simulink library "bpm_blower_propulsion_module_lib"  (R2015b)
settings: Solver=ode45  StartTime=0.0  StopTime=10.0  RelTol=1e-3
values from neighbouring files (symbols this model uses):
  bpm_imp_cmd_filt_den = single(1.0)    [bpm_blower_propulsion_module_init.m]
  bpm_imp_cmd_filt_num = single(1.0)    [bpm_blower_propulsion_module_init.m]
  bpm_imp_ctl_filt_n = single(1.0)    [bpm_blower_propulsion_module_init.m]
  bpm_imp_ctl_kd = single(0.001)    [bpm_blower_propulsion_module_init.m]
  bpm_imp_ctl_ki = single(0.40)    [bpm_blower_propulsion_module_init.m]
  bpm_imp_ctl_kp = single(0.015)    [bpm_blower_propulsion_module_init.m]
  bpm_imp_ctl_ts = 0.016    [bpm_blower_propulsion_module_init.m]
  bpm_imp_max_voltage = single(16.6)    [bpm_blower_propulsion_module_init.m]
  bpm_imp_motor_friction_coeff = bpm_imp_noload_curr*bpm_imp_motor_torque_k/bpm_imp_noload_speed    [bpm_blower_propulsion_module_prep.m]
  bpm_imp_motor_r = single(1.2)    [bpm_blower_propulsion_module_init.m]
  bpm_imp_motor_speed_k = single(374*2*pi/60)    [bpm_blower_propulsion_module_init.m]
  bpm_imp_motor_torque_k = single(0.0255)    [bpm_blower_propulsion_module_init.m]
  bpm_imp_speed_filt_den = single(1.0)    [bpm_blower_propulsion_module_init.m]
  bpm_imp_speed_filt_num = single(1.0)    [bpm_blower_propulsion_module_init.m]
  bpm_sensor_delay = 1    [bpm_blower_propulsion_module_init.m]
  bpm_sensor_rand_seed = 1337    [bpm_blower_propulsion_module_init.m]
  bpm_sensor_sf = single(1)    [bpm_blower_propulsion_module_init.m]
  bpm_sensor_sigma_u = .00001    (= 1e-05)    [bpm_blower_propulsion_module_init.m]
  bpm_sensor_sigma_v = .00001    (= 1e-05)    [bpm_blower_propulsion_module_init.m]
  bpm_servo_ctl_filt_n = single(1.0)    [bpm_blower_propulsion_module_init.m]
  bpm_servo_ctl_kd = single(0.8)    [bpm_blower_propulsion_module_init.m]
  bpm_servo_ctl_ki = single(1.5)    [bpm_blower_propulsion_module_init.m]
  bpm_servo_ctl_kp = single(5.0)    [bpm_blower_propulsion_module_init.m]
  bpm_servo_ctl_ts = 0.016    [bpm_blower_propulsion_module_init.m]
  bpm_servo_max_theta = abp_nozzle_gear_ratio*(abp_nozzle_max_open_angle - abp_nozzle_min_open_angle)    [bpm_blower_propulsion_module_prep.m]
  bpm_servo_max_voltage = single(6)    [bpm_blower_propulsion_module_init.m]
  bpm_servo_min_theta = 0    [bpm_blower_propulsion_module_prep.m]
  bpm_servo_motor_friction_coeff = single(0.0000003)    [bpm_blower_propulsion_module_init.m]
  bpm_servo_motor_gear_box_inertia = single(.000000025)    [bpm_blower_propulsion_module_init.m]
  bpm_servo_motor_gear_ratio = single(1/100)    [bpm_blower_propulsion_module_init.m]
  bpm_servo_motor_k = bpm_servo_peak_torque*bpm_servo_motor_gear_ratio/(bpm_servo_peak_curr)    [bpm_blower_propulsion_module_prep.m]
  bpm_servo_motor_r = bpm_servo_max_voltage/bpm_servo_peak_curr    [bpm_blower_propulsion_module_prep.m]
  bpm_servo_pwm2angle = (bpm_servo_max_theta-bpm_servo_min_theta)/(abp_servo_max_PWM-abp_servo_min_PWM)    [bpm_blower_propulsion_module_prep.m]
  bpm_servo_pwm2angle_bias = bpm_servo_min_theta/bpm_servo_pwm2angle - abp_servo_min_PWM    [bpm_blower_propulsion_module_prep.m]
undefined symbols (not defined in the file or in its folder): astrobee_time_step_size, bpm_blower_speed2pwm, bpm_nozzle_gear_ratio, DiscIntNeverNeededParam
libraries: bpm_common_lib x4, simulink x3, util_common_lib x1
settings Model: Creator=rhnakamu  LastModifiedBy=jfusco1
settings DataIOCC: SaveFormat=Array
settings HardwareCC: ProdBitPerPointer=32  ProdLargestAtomicFloat=None  ProdIntDivRoundTo=Undefined  ProdEndianess=Unspecified  ProdWordSize=32  ProdHWDeviceType=32-bit Generic
settings GRTTargetCC: GeneratePreprocessorConditionals=Disable all
settings ConfigComp: CovModelRefEnable=Off

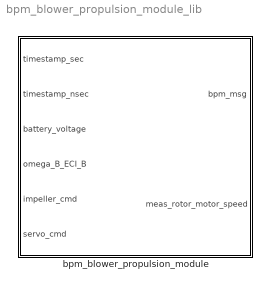
== system bpm_blower_propulsion_module_lib ==
  bpm_blower_propulsion_module : Subsystem

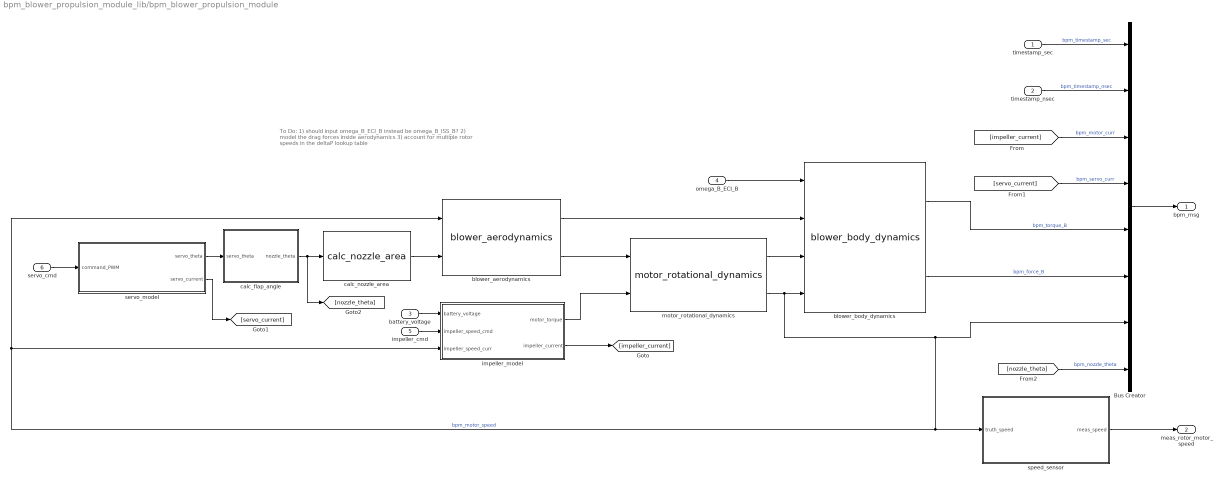
== system bpm_blower_propulsion_module_lib/bpm_blower_propulsion_module ==
  note: To Do:
      | 	1) should input omega_B_ECI_B instead be omega_B_ISS_B?
      | 	2) model the drag forces inside aerodynamics
      | 	3) account for multiple rotor speeds in the deltaP lookup table
  timestamp_sec : Inport
  timestamp_nsec : Inport  Port=2
  battery_voltage : Inport  Port=3
  omega_B_ECI_B : Inport  Port=4
  impeller_cmd : Inport  Port=5
  servo_cmd : Inport  Port=6
  Bus Creator : BusCreator  Inputs=8  OutDataTypeStr=Bus: bpm_msg  NonVirtualBus=on
      settings: InheritFromInputs=off
  blower_aerodynamics : bpm_common_lib/blower_aerodynamics  VariantControl=blw_blower_algebraic == true
  blower_body_dynamics : bpm_common_lib/blower_body_dynamics
  calc_flap_angle : Subsystem
  calc_nozzle_area : bpm_common_lib/calc_nozzle_area
  impeller_model : Subsystem
  motor_rotational_dynamics : bpm_common_lib/motor_rotational_dynamics
  servo_model : Subsystem  TreatAsAtomicUnit=on
  speed_sensor : Subsystem
  bpm_msg : Outport
  meas_rotor_motor_speed : Outport  Port=2
  wires:
  timestamp_sec/1 -> Bus Creator/1  "bpm_timestamp_sec"
  timestamp_nsec/1 -> Bus Creator/2  "bpm_timestamp_nsec"
  [nozzle_theta] -> Bus Creator/8  "bpm_nozzle_theta"
  blower_aerodynamics/1 -> blower_body_dynamics/2
  battery_voltage/1 -> impeller_model/1(battery_voltage)
  servo_model/1(servo_theta) -> calc_flap_angle/1(servo_theta)
  calc_nozzle_area/1 -> blower_aerodynamics/2
  motor_rotational_dynamics/2 -> blower_body_dynamics/4, blower_aerodynamics/1, impeller_model/3(impeller_speed_curr), speed_sensor/1(truth_speed), Bus Creator/7  "bpm_motor_speed"
  servo_model/2(servo_current) -> [servo_current]
  blower_body_dynamics/1 -> Bus Creator/5  "bpm_torque_B"
  blower_body_dynamics/2 -> Bus Creator/6  "bpm_force_B"
  speed_sensor/1(meas_speed) -> meas_rotor_motor_speed/1
  omega_B_ECI_B/1 -> blower_body_dynamics/1
  servo_cmd/1 -> servo_model/1(command_PWM)
  impeller_cmd/1 -> impeller_model/2(impeller_speed_cmd)
  impeller_model/1(motor_torque) -> motor_rotational_dynamics/2
  impeller_model/2(impeller_current) -> [impeller_current]
  [servo_current] -> Bus Creator/4  "bpm_servo_curr"
  [impeller_current] -> Bus Creator/3  "bpm_motor_curr"
  Bus Creator/1 -> bpm_msg/1
  calc_flap_angle/1(nozzle_theta) -> [nozzle_theta], calc_nozzle_area/1
  blower_aerodynamics/2 -> motor_rotational_dynamics/1
  motor_rotational_dynamics/1 -> blower_body_dynamics/3

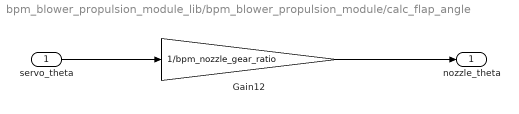
== system bpm_blower_propulsion_module_lib/bpm_blower_propulsion_module/calc_flap_angle ==
  servo_theta : Inport
  Gain12 : Gain  Gain=1/bpm_nozzle_gear_ratio
  nozzle_theta : Outport
  wires:
  servo_theta/1 -> Gain12/1
  Gain12/1 -> nozzle_theta/1

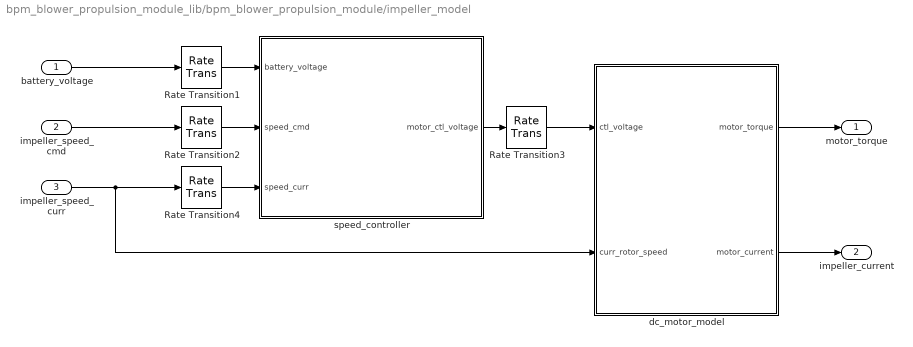
== system bpm_blower_propulsion_module_lib/bpm_blower_propulsion_module/impeller_model ==
  battery_voltage : Inport
  impeller_speed_cmd : Inport  Port=2
  impeller_speed_curr : Inport  Port=3
  Rate Transition{1..4} (4 alike) : RateTransition
      settings: AttributesFormatString=sampleTime: %<OutPortSampleTime>
  dc_motor_model : Subsystem  TreatAsAtomicUnit=on
  speed_controller : Subsystem  TreatAsAtomicUnit=on
  motor_torque : Outport
  impeller_current : Outport  Port=2
  wires:
  impeller_speed_cmd/1 -> Rate Transition2/1
  Rate Transition4/1 -> speed_controller/3(speed_curr)
  Rate Transition2/1 -> speed_controller/2(speed_cmd)
  Rate Transition1/1 -> speed_controller/1(battery_voltage)
  Rate Transition3/1 -> dc_motor_model/1(ctl_voltage)
  battery_voltage/1 -> Rate Transition1/1
  dc_motor_model/2(motor_current) -> impeller_current/1
  speed_controller/1(motor_ctl_voltage) -> Rate Transition3/1
  dc_motor_model/1(motor_torque) -> motor_torque/1
  impeller_speed_curr/1 -> dc_motor_model/2(curr_rotor_speed), Rate Transition4/1

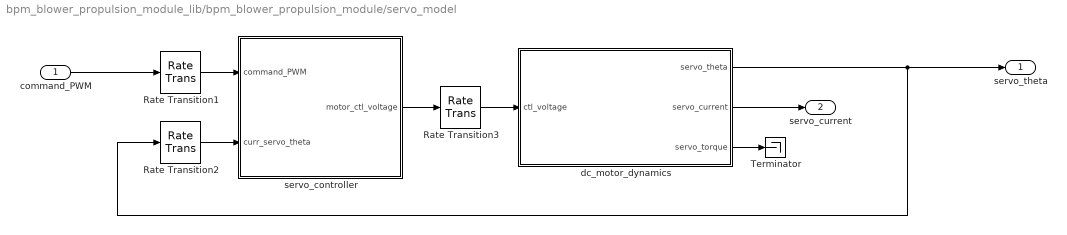
== system bpm_blower_propulsion_module_lib/bpm_blower_propulsion_module/servo_model ==
  command_PWM : Inport
  Rate Transition1 : RateTransition
      settings: AttributesFormatString=sampleTime: %<OutPortSampleTime>
  Rate Transition2 : RateTransition
      settings: AttributesFormatString=sampleTime: %<OutPortSampleTime>
  Rate Transition3 : RateTransition
      settings: AttributesFormatString=sampleTime: %<OutPortSampleTime>
  Terminator : Terminator
  dc_motor_dynamics : Subsystem
  servo_controller : Subsystem
  servo_theta : Outport
  servo_current : Outport  Port=2
  wires:
  dc_motor_dynamics/3(servo_torque) -> Terminator/1
  command_PWM/1 -> Rate Transition1/1
  servo_controller/1(motor_ctl_voltage) -> Rate Transition3/1
  Rate Transition3/1 -> dc_motor_dynamics/1(ctl_voltage)
  Rate Transition1/1 -> servo_controller/1(command_PWM)
  Rate Transition2/1 -> servo_controller/2(curr_servo_theta)
  dc_motor_dynamics/2(servo_current) -> servo_current/1
  dc_motor_dynamics/1(servo_theta) -> servo_theta/1, Rate Transition2/1

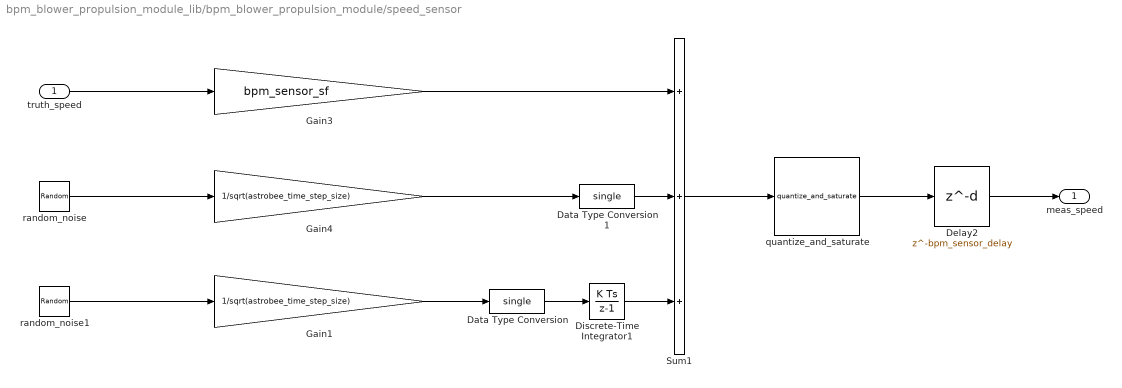
== system bpm_blower_propulsion_module_lib/bpm_blower_propulsion_module/speed_sensor ==
  truth_speed : Inport
  Data Type Conversion : DataTypeConversion  OutDataTypeStr=single
  Data Type Conversion1 : DataTypeConversion  OutDataTypeStr=single
  Delay2 : Delay  DelayLength=bpm_sensor_delay
      settings: AttributesFormatString=|
      | IC: %<InitialCondition>
      | Delay: %<DelayLength>
  Discrete-Time Integrator1 : DiscreteIntegrator  InitialCondition=single(0)  InitialConditionSetting=State (most efficient)  SampleTime=-1  ICPrevOutput=DiscIntNeverNeededParam  ICPrevScaledInput=DiscIntNeverNeededParam
      settings: AttributesFormatString=IC:%<InitialCondition>
  Gain1 : Gain  Gain=1/sqrt(astrobee_time_step_size)
  Gain3 : Gain  Gain=bpm_sensor_sf
  Gain4 : Gain  Gain=1/sqrt(astrobee_time_step_size)
  Sum1 : Sum  Inputs=+++
  quantize_and_saturate : util_common_lib/quantize_and_saturate  RES=bpm_sensor_resolution  OPER=truncate  out_min=bpm_sensor_min  out_max=bpm_sensor_max
      settings: AttributesFormatString=|
      | Resolution: %<RES>
      | Max: %<out_max>
      | Min: %<out_min>
  random_noise : RandomNumber  Variance=bpm_sensor_sigma_u.^2  Seed=bpm_sensor_rand_seed  SampleTime=astrobee_time_step_size
      settings: AttributesFormatString=|
      | Variance:%<Variance>
      | Mean:%<Mean>
      | Seed:%<Seed>
      | Sample Time:%<SampleTime>
  random_noise1 : RandomNumber  Variance=bpm_sensor_sigma_v.^2  Seed=bpm_sensor_rand_seed+1  SampleTime=astrobee_time_step_size
      settings: AttributesFormatString=|
      | Variance:%<Variance>
      | Mean:%<Mean>
      | Seed:%<Seed>
      | Sample Time:%<SampleTime>
  meas_speed : Outport
  wires:
  Data Type Conversion/1 -> Discrete-Time Integrator1/1
  Gain3/1 -> Sum1/1
  Data Type Conversion1/1 -> Sum1/2
  Discrete-Time Integrator1/1 -> Sum1/3
  Sum1/1 -> quantize_and_saturate/1
  Gain4/1 -> Data Type Conversion1/1
  Gain1/1 -> Data Type Conversion/1
  random_noise1/1 -> Gain1/1
  random_noise/1 -> Gain4/1
  truth_speed/1 -> Gain3/1
  quantize_and_saturate/1 -> Delay2/1
  Delay2/1 -> meas_speed/1

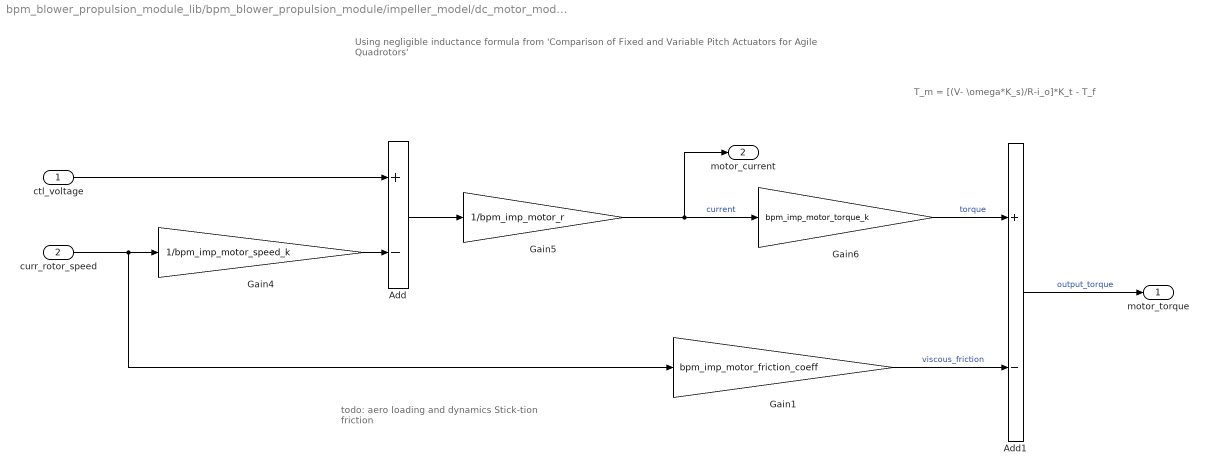
== system bpm_blower_propulsion_module_lib/bpm_blower_propulsion_module/impeller_model/dc_motor_model ==
  note: todo:
      | aero loading and dynamics
      | Stick-tion friction
  note: Using negligible inductance formula from 'Comparison of Fixed and Variable Pitch Actuators for Agile Quadrotors'
  note: T_m = [(V- \omega*K_s)/R-i_o]*K_t - T_f
  ctl_voltage : Inport
  curr_rotor_speed : Inport  Port=2
  Add : Sum  Inputs=+-
  Add1 : Sum  Inputs=+-
  Gain1 : Gain  Gain=bpm_imp_motor_friction_coeff
  Gain4 : Gain  Gain=1/bpm_imp_motor_speed_k
  Gain5 : Gain  Gain=1/bpm_imp_motor_r
  Gain6 : Gain  Gain=bpm_imp_motor_torque_k
  motor_torque : Outport
  motor_current : Outport  Port=2
  wires:
  Gain5/1 -> Gain6/1, motor_current/1  "current"
  ctl_voltage/1 -> Add/1
  Gain4/1 -> Add/2
  curr_rotor_speed/1 -> Gain1/1, Gain4/1
  Add/1 -> Gain5/1
  Gain6/1 -> Add1/1  "torque"
  Add1/1 -> motor_torque/1  "output_torque"
  Gain1/1 -> Add1/2  "viscous_friction"

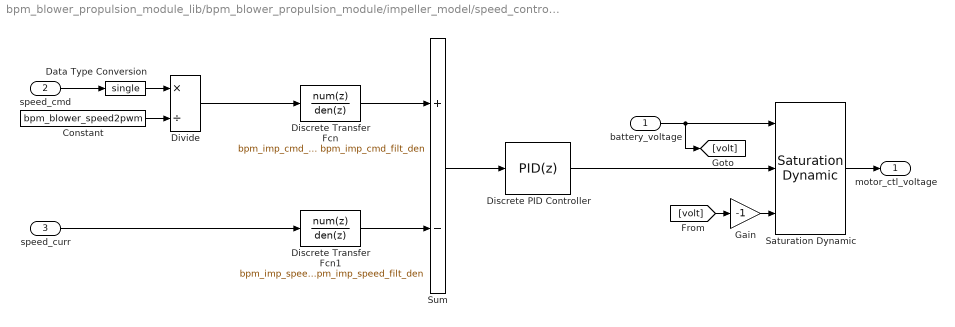
== system bpm_blower_propulsion_module_lib/bpm_blower_propulsion_module/impeller_model/speed_controller ==
  battery_voltage : Inport
  speed_cmd : Inport  Port=2
  speed_curr : Inport  Port=3
  Constant : Constant  Value=bpm_blower_speed2pwm
  Data Type Conversion : DataTypeConversion  OutDataTypeStr=single
  Discrete Transfer Fcn : DiscreteTransferFcn  Numerator=bpm_imp_cmd_filt_num  Denominator=bpm_imp_cmd_filt_den  SampleTime=bpm_imp_ctl_ts
      settings: AttributesFormatString=|
      | Num: %<Numerator>
      | Den: %<Denominator>
      | TS: %<SampleTime>
  Discrete Transfer Fcn1 : DiscreteTransferFcn  Numerator=bpm_imp_speed_filt_num  Denominator=bpm_imp_speed_filt_den  SampleTime=bpm_imp_ctl_ts
      settings: AttributesFormatString=|
      | Num: %<Numerator>
      | Den: %<Denominator>
      | TS: %<SampleTime>
  Discrete PID Controller : simulink/Continuous/PID Controller  Controller=PID  TimeDomain=Discrete-time  SampleTime=bpm_imp_ctl_ts  IntegratorMethod=Forward Euler  FilterMethod=Forward Euler  Form=Parallel  UseFilter=on  ControllerParametersSource=internal  P=bpm_imp_ctl_kp  I=bpm_imp_ctl_ki  D=bpm_imp_ctl_kd  N=bpm_imp_ctl_filt_n  InitialConditionSource=internal  InitialConditionForIntegrator=0  InitialConditionForFilter=0  ExternalReset=none  LimitOutput=on  UpperSaturationLimit=bpm_imp_max_voltage  LowerSaturationLimit=-bpm_imp_max_voltage  LinearizeAsGain=off  AntiWindupMode=clamping  Kb=1  TrackingMode=off  Kt=1  PParamMin=[]  PParamMax=[]  IParamMin=[]  IParamMax=[]  DParamMin=[]  DParamMax=[]  NParamMin=[]  NParamMax=[]  KbParamMin=[]  KbParamMax=[]  KtParamMin=[]  KtParamMax=[]  POutMin=[]  POutMax=[]  IOutMin=[]  IOutMax=[]  DOutMin=[]  DOutMax=[]  NOutMin=[]  NOutMax=[]  KbOutMin=[]  KbOutMax=[]  KtOutMin=[]  KtOutMax=[]  IntegratorOutMin=[]  IntegratorOutMax=[]  FilterOutMin=[]  FilterOutMax=[]  SumOutMin=[]  SumOutMax=[]  SumI1OutMin=[]  SumI1OutMax=[]  SumI2OutMin=[]  SumI2OutMax=[]  SumI3OutMin=[]  SumI3OutMax=[]  SumDOutMin=[]  SumDOutMax=[]  SaturationOutMin=[]  SaturationOutMax=[]  IntegratorContinuousStateAttributes=''  IntegratorStateMustResolveToSignalObject=off  IntegratorRTWStateStorageClass=Auto  FilterContinuousStateAttributes=''  FilterStateMustResolveToSignalObject=off  FilterRTWStateStorageClass=Auto  DifferentiatorICPrevScaledInput=0  DifferentiatorOutMin=[]  DifferentiatorOutMax=[]
      settings: AttributesFormatString=|
      | Kp: %<P>
      | Ki: %<I>
      | Kd: %<D>
      | NFilt: %<N>
      | Ts: %<SampleTime>
      | 
      | min: %<LowerSaturationLimit>
      | max: %<UpperSaturationLimit>
  Divide : Product  Inputs=*/
  Gain : Gain  Gain=-1
  Saturation Dynamic : simulink/Discontinuities/Saturation Dynamic  OutMin=[]  OutMax=[]  OutDataTypeStr=Inherit: Same as second input  OutDataType=fixdt(1, 16)  OutScaling=2^-10  DoSatur=off
  Sum : Sum  Inputs=+-
  motor_ctl_voltage : Outport
  wires:
  Gain/1 -> Saturation Dynamic/3
  [volt] -> Gain/1
  Discrete PID Controller/1 -> Saturation Dynamic/2
  battery_voltage/1 -> [volt], Saturation Dynamic/1
  speed_curr/1 -> Discrete Transfer Fcn1/1
  Sum/1 -> Discrete PID Controller/1
  Saturation Dynamic/1 -> motor_ctl_voltage/1
  Discrete Transfer Fcn1/1 -> Sum/2
  Discrete Transfer Fcn/1 -> Sum/1
  speed_cmd/1 -> Data Type Conversion/1
  Divide/1 -> Discrete Transfer Fcn/1
  Constant/1 -> Divide/2
  Data Type Conversion/1 -> Divide/1

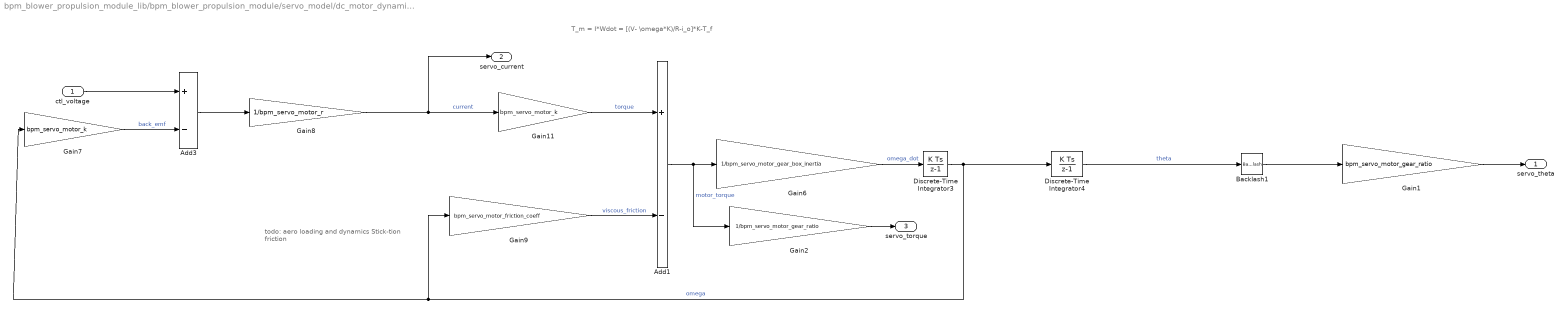
== system bpm_blower_propulsion_module_lib/bpm_blower_propulsion_module/servo_model/dc_motor_dynamics ==
  note: T_m = I*Wdot = [(V- \omega*K)/R-i_o]*K-T_f
  note: todo:
      | aero loading and dynamics
      | Stick-tion friction
  ctl_voltage : Inport
  Add1 : Sum  Inputs=+-
  Add3 : Sum  Inputs=+-
  Backlash1 : Backlash  BacklashWidth=bpm_servo_motor_backlash_deadband
      settings: AttributesFormatString=width: %<BacklashWidth>
  Discrete-Time Integrator3 : DiscreteIntegrator  InitialCondition=single(0)  SampleTime=-1  ICPrevOutput=DiscIntNeverNeededParam  ICPrevScaledInput=DiscIntNeverNeededParam
      settings: AttributesFormatString=IC: %<InitialCondition>
  Discrete-Time Integrator4 : DiscreteIntegrator  InitialCondition=bpm_servo_min_theta/bpm_servo_motor_gear_ratio  SampleTime=-1  LimitOutput=on  UpperSaturationLimit=bpm_servo_max_theta/bpm_servo_motor_gear_ratio  LowerSaturationLimit=bpm_servo_min_theta/bpm_servo_motor_gear_ratio  ICPrevOutput=DiscIntNeverNeededParam  ICPrevScaledInput=DiscIntNeverNeededParam
      settings: AttributesFormatString=|
      | IC: %<InitialCondition>
      | max: %<UpperSaturationLimit>
      | min: %<LowerSaturationLimit>
  Gain1 : Gain  Gain=bpm_servo_motor_gear_ratio
  Gain11 : Gain  Gain=bpm_servo_motor_k
  Gain2 : Gain  Gain=1/bpm_servo_motor_gear_ratio
  Gain6 : Gain  Gain=1/bpm_servo_motor_gear_box_inertia
  Gain7 : Gain  Gain=bpm_servo_motor_k
  Gain8 : Gain  Gain=1/bpm_servo_motor_r
  Gain9 : Gain  Gain=bpm_servo_motor_friction_coeff
  servo_theta : Outport
  servo_current : Outport  Port=2
  servo_torque : Outport  Port=3
  wires:
  ctl_voltage/1 -> Add3/1
  Gain2/1 -> servo_torque/1
  Gain9/1 -> Add1/2  "viscous_friction"
  Gain11/1 -> Add1/1  "torque"
  Add1/1 -> Gain2/1, Gain6/1  "motor_torque"
  Gain1/1 -> servo_theta/1
  Backlash1/1 -> Gain1/1
  Discrete-Time Integrator3/1 -> Gain9/1, Gain7/1, Discrete-Time Integrator4/1  "omega"
  Discrete-Time Integrator4/1 -> Backlash1/1  "theta"
  Gain8/1 -> servo_current/1, Gain11/1  "current"
  Add3/1 -> Gain8/1
  Gain7/1 -> Add3/2  "back_emf"
  Gain6/1 -> Discrete-Time Integrator3/1  "omega_dot"

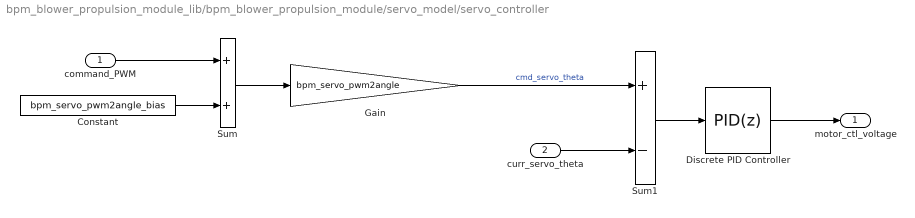
== system bpm_blower_propulsion_module_lib/bpm_blower_propulsion_module/servo_model/servo_controller ==
  command_PWM : Inport
  curr_servo_theta : Inport  Port=2
  Constant : Constant  Value=bpm_servo_pwm2angle_bias
  Discrete PID Controller : simulink/Continuous/PID Controller  Controller=PID  TimeDomain=Discrete-time  SampleTime=bpm_servo_ctl_ts  IntegratorMethod=Forward Euler  FilterMethod=Forward Euler  Form=Parallel  UseFilter=on  ControllerParametersSource=internal  P=bpm_servo_ctl_kp  I=bpm_servo_ctl_ki  D=bpm_servo_ctl_kd  N=bpm_servo_ctl_filt_n  InitialConditionSource=internal  InitialConditionForIntegrator=0  InitialConditionForFilter=0  ExternalReset=none  LimitOutput=on  UpperSaturationLimit=bpm_servo_max_voltage  LowerSaturationLimit=-bpm_servo_max_voltage  LinearizeAsGain=off  AntiWindupMode=clamping  Kb=1  TrackingMode=off  Kt=1  PParamMin=[]  PParamMax=[]  IParamMin=[]  IParamMax=[]  DParamMin=[]  DParamMax=[]  NParamMin=[]  NParamMax=[]  KbParamMin=[]  KbParamMax=[]  KtParamMin=[]  KtParamMax=[]  POutMin=[]  POutMax=[]  IOutMin=[]  IOutMax=[]  DOutMin=[]  DOutMax=[]  NOutMin=[]  NOutMax=[]  KbOutMin=[]  KbOutMax=[]  KtOutMin=[]  KtOutMax=[]  IntegratorOutMin=[]  IntegratorOutMax=[]  FilterOutMin=[]  FilterOutMax=[]  SumOutMin=[]  SumOutMax=[]  SumI1OutMin=[]  SumI1OutMax=[]  SumI2OutMin=[]  SumI2OutMax=[]  SumI3OutMin=[]  SumI3OutMax=[]  SumDOutMin=[]  SumDOutMax=[]  SaturationOutMin=[]  SaturationOutMax=[]  IntegratorContinuousStateAttributes=''  IntegratorStateMustResolveToSignalObject=off  IntegratorRTWStateStorageClass=Auto  FilterContinuousStateAttributes=''  FilterStateMustResolveToSignalObject=off  FilterRTWStateStorageClass=Auto  DifferentiatorICPrevScaledInput=0  DifferentiatorOutMin=[]  DifferentiatorOutMax=[]
      settings: AttributesFormatString=|
      | Kp: %<P>
      | Ki: %<I>
      | Kd: %<D>
      | NFilt: %<N>
      | Ts: %<SampleTime>
      | 
      | Min: %<LowerSaturationLimit>
      | Max: %<UpperSaturationLimit>
  Gain : Gain  Gain=bpm_servo_pwm2angle
  Sum : Sum
  Sum1 : Sum  Inputs=+-
  motor_ctl_voltage : Outport
  wires:
  Sum/1 -> Gain/1
  Sum1/1 -> Discrete PID Controller/1
  command_PWM/1 -> Sum/1
  Constant/1 -> Sum/2
  Discrete PID Controller/1 -> motor_ctl_voltage/1
  curr_servo_theta/1 -> Sum1/2
  Gain/1 -> Sum1/1  "cmd_servo_theta"
